simulink model "Vergleich_linear_nichtlinear"  (R2021b)
settings: Solver=FixedStepAuto  StartTime=0.0  StopTime=10  FixedStep=1/1e4  RelTol=1e-3
undefined symbols (not defined in the file): A, B, C, start_deg, V_m, V_m_dyn, x_c
settings Model: Creator=basti  LastModifiedBy=basti

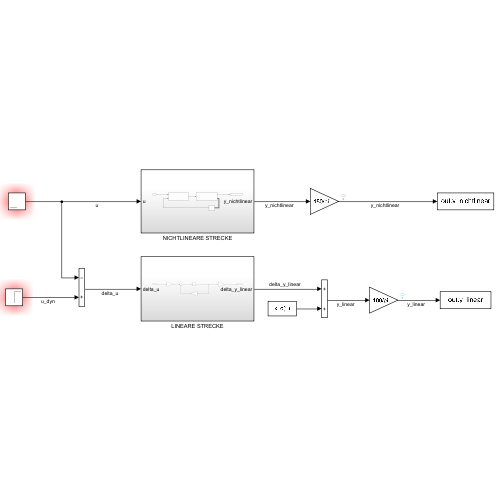
[thumbnail: Simulink's stored preview of the top-level diagram]
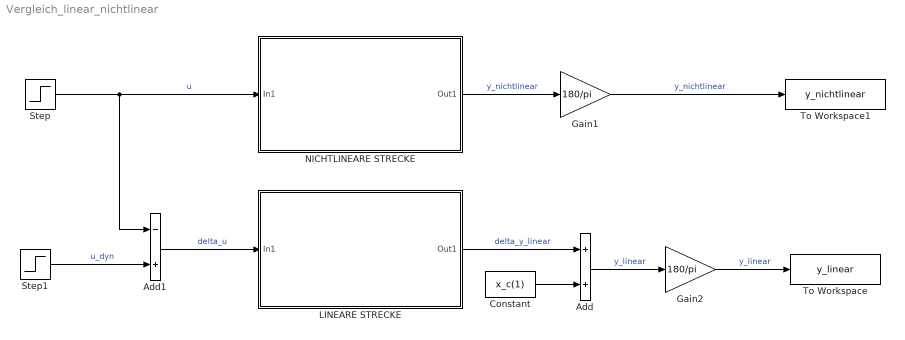
== system Vergleich_linear_nichtlinear ==
  Add : Sum
  Add1 : Sum  Inputs=-+
  Constant : Constant  Value=x_c(1)
  Gain1 : Gain  Gain=180/pi
  Gain2 : Gain  Gain=180/pi
  LINEARE STRECKE : Subsystem
  NICHTLINEARE STRECKE : Subsystem
  Step : Step  Time=0  After=V_m  SampleTime=0
  Step1 : Step  Time=0  After=V_m_dyn  SampleTime=0
  To Workspace : ToWorkspace  VariableName=y_linear  SaveFormat=Timeseries  SampleTime=-1
  To Workspace1 : ToWorkspace  VariableName=y_nichtlinear  SaveFormat=Timeseries  SampleTime=-1
  wires:
  LINEARE STRECKE/1(Out1) -> Add/1  "delta_y_linear"
  NICHTLINEARE STRECKE/1(Out1) -> Gain1/1  "y_nichtlinear"
  Constant/1 -> Add/2
  Add/1 -> Gain2/1  "y_linear"
  Step/1 -> Add1/1, NICHTLINEARE STRECKE/1(In1)  "u"
  Gain2/1 -> To Workspace/1  "y_linear"
  Gain1/1 -> To Workspace1/1  "y_nichtlinear"
  Add1/1 -> LINEARE STRECKE/1(In1)  "delta_u"
  Step1/1 -> Add1/2  "u_dyn"

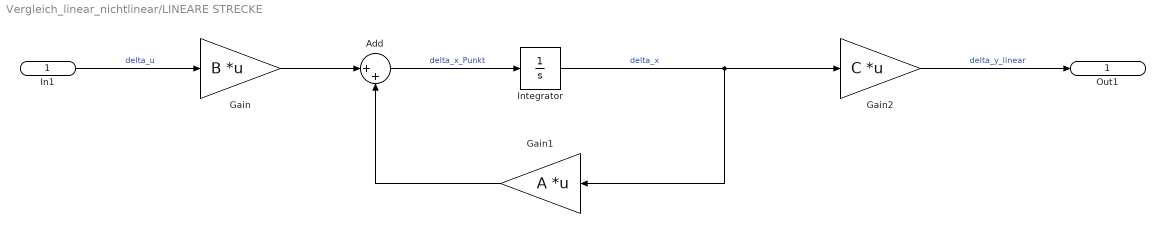
== system Vergleich_linear_nichtlinear/LINEARE STRECKE ==
  In1 : Inport
  Add : Sum  Inputs=|++
  Gain : Gain  Gain=B  Multiplication=Matrix(K*u) (u vector)
  Gain1 : Gain  Gain=A  Multiplication=Matrix(K*u) (u vector)
  Gain2 : Gain  Gain=C  Multiplication=Matrix(K*u) (u vector)
  Integrator : Integrator  InitialCondition=[(start_deg*pi/180); 0; 0; 0]
  Out1 : Outport
  wires:
  Gain/1 -> Add/1
  Integrator/1 -> Gain2/1, Gain1/1  "delta_x"
  Add/1 -> Integrator/1  "delta_x_Punkt"
  Gain1/1 -> Add/2
  In1/1 -> Gain/1  "delta_u"
  Gain2/1 -> Out1/1  "delta_y_linear"

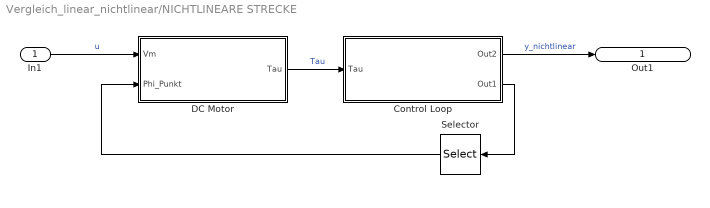
== system Vergleich_linear_nichtlinear/NICHTLINEARE STRECKE ==
  In1 : Inport
  Control Loop : Subsystem
  DC Motor : Subsystem
  Selector : Selector  InputPortWidth=4  IndexOptions=Index vector (dialog)  Indices=4  OutputSizes=1
  Out1 : Outport
  wires:
  Control Loop/1(Out2) -> Out1/1  "y_nichtlinear"
  In1/1 -> DC Motor/1(Vm)  "u"
  DC Motor/1(Tau) -> Control Loop/1(Tau)  "Tau"
  Control Loop/2(Out1) -> Selector/1
  Selector/1 -> DC Motor/2(Phi_Punkt)

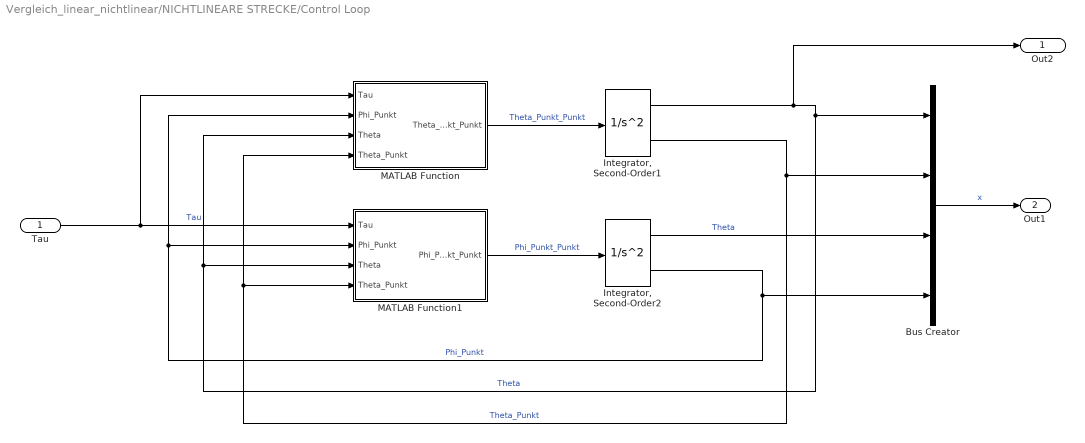
== system Vergleich_linear_nichtlinear/NICHTLINEARE STRECKE/Control Loop ==
  Tau : Inport
  Bus Creator : BusCreator  Inputs=4
  "Integrator, Second-Order1" : SecondOrderIntegrator  ICX=x_c(1)+(start_deg*pi/180)  ICDXDT=x_c(2)
  "Integrator, Second-Order2" : SecondOrderIntegrator  ICX=x_c(3)  ICDXDT=x_c(4)
  MATLAB Function : MATLAB Function  TreatAsAtomicUnit=on
  MATLAB Function1 : MATLAB Function  TreatAsAtomicUnit=on
  Out2 : Outport
  Out1 : Outport  Port=2
  wires:
  MATLAB Function/1(Theta_Punkt_Punkt) -> "Integrator, Second-Order1"/1  "Theta_Punkt_Punkt"
  MATLAB Function1/1(Phi_Punkt_Punkt) -> "Integrator, Second-Order2"/1  "Phi_Punkt_Punkt"
  "Integrator, Second-Order2"/2 -> MATLAB Function1/2(Phi_Punkt), MATLAB Function/2(Phi_Punkt), Bus Creator/4  "Phi_Punkt"
  "Integrator, Second-Order1"/1 -> Out2/1, MATLAB Function1/3(Theta), MATLAB Function/3(Theta), Bus Creator/1  "Theta"
  "Integrator, Second-Order1"/2 -> MATLAB Function/4(Theta_Punkt), MATLAB Function1/4(Theta_Punkt), Bus Creator/2  "Theta_Punkt"
  Tau/1 -> MATLAB Function/1(Tau), MATLAB Function1/1(Tau)  "Tau"
  "Integrator, Second-Order2"/1 -> Bus Creator/3  "Theta"
  Bus Creator/1 -> Out1/1  "x"

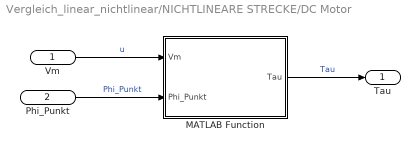
== system Vergleich_linear_nichtlinear/NICHTLINEARE STRECKE/DC Motor ==
  Vm : Inport
  Phi_Punkt : Inport  Port=2
  MATLAB Function : MATLAB Function  TreatAsAtomicUnit=on
  Tau : Outport
  wires:
  Vm/1 -> MATLAB Function/1(Vm)  "u"
  Phi_Punkt/1 -> MATLAB Function/2(Phi_Punkt)  "Phi_Punkt"
  MATLAB Function/1(Tau) -> Tau/1  "Tau"

== matlab function Vergleich_linear_nichtlinear/NICHTLINEARE STRECKE/Control Loop/MATLAB Function1 ==
  data: Tau input; Phi_Punkt_Punkt output; Phi_Punkt input; Theta input; Theta_Punkt input
function Phi_Punkt_Punkt = fcn(Tau, Phi_Punkt, Theta, Theta_Punkt)
    % Konstanten aufrufen
    c = Konstanten();
    
    % Berechnung
    Phi_Punkt_Punkt = (((c.m1*c.l1+c.m2*c.l2)*c.g*sin(Theta)-c.c1*Theta_Punkt-(c.m1*c.l1^2+c.m2*c.l2^2+c.J1+c.J2)*(Tau-c.c2*Phi_Punkt)/c.J2)/c.J2)/(1-(c.m1*c.l1^2+c.m2*c.l2^2+c.J1+c.J2)/c.J2);

== matlab function Vergleich_linear_nichtlinear/NICHTLINEARE STRECKE/Control Loop/MATLAB Function ==
  data: Tau input; Theta_Punkt_Punkt output; Phi_Punkt input; Theta input; Theta_Punkt input
function Theta_Punkt_Punkt = fcn(Tau, Phi_Punkt, Theta, Theta_Punkt)
    % Konstanten aufrufen
    c = Konstanten();
    
    % Berechnung
    Theta_Punkt_Punkt = ((Tau-c.c2*Phi_Punkt-(c.m1*c.l1+c.m2*c.l2)*c.g*sin(Theta)+c.c1*Theta_Punkt)/c.J2)/(1-(c.m1*c.l1^2+c.m2*c.l2^2+c.J1+c.J2)/c.J2);

== matlab function Vergleich_linear_nichtlinear/NICHTLINEARE STRECKE/DC Motor/MATLAB Function ==
  data: Vm input; Tau output; Phi_Punkt input
function Tau = fcn(Vm, Phi_Punkt)
    % Konstanten
    c = Konstanten();
    
    % Berechnung
    Tau = c.Kt*(Vm-c.Kb*Phi_Punkt)/c.Ra;
